simulink model "HighpassFilteredAccelerometer"  (R2019b)
settings: Solver=FixedStepAuto  StartTime=0.0  StopTime=10  FixedStep=1e-5  RelTol=1e-3
model workspace (MAT data in the model file):
  DC_Noise_Amplitude = 0.45
libraries: dsparch4 x12, simulink x9, powerlib x2
settings Model: EnablePacing=on  Creator=HUAWEI  LastModifiedBy=19398
settings DataIOCC: ReturnWorkspaceOutputs=off
settings OptimizationCC: DefaultParameterBehavior=Inlined  EnhancedBackFolding=on  PassReuseOutputArgsAs=Individual arguments  ZeroExternalMemoryAtStartup=off  ZeroInternalMemoryAtStartup=off  OptimizeBlockOrder=speed  DifferentSizesBufferReuse=on  OptimizationCustomize=off  EfficientTunableParamExpr=on
settings DebuggingCC: ParameterTunabilityLossMsg=error
settings SFSimCC: MATLABDynamicMemAlloc=off
settings RTWCC: SystemTargetFile=ert.tlc  TemplateMakefile=ert_default_tmf  GenerateReport=on  IncludeHyperlinkInReport=on  LaunchReport=on  GenerateTraceInfo=on  GenerateTraceReport=on  GenerateTraceReportSl=on  GenerateTraceReportSf=on  GenerateTraceReportEml=on
settings CodeAppCC: ForceParamTrailComments=on  IgnoreCustomStorageClasses=off  OperatorAnnotations=on  SimulinkDataObjDesc=on  SFDataObjDesc=on  InsertBlockDesc=on
settings ERTTargetCC: TargetLangStandard=C99 (ISO)  GenerateSampleERTMain=on  InlinedParameterPlacement=NonHierarchical  ERTCustomFileTemplate=example_file_process.tlc

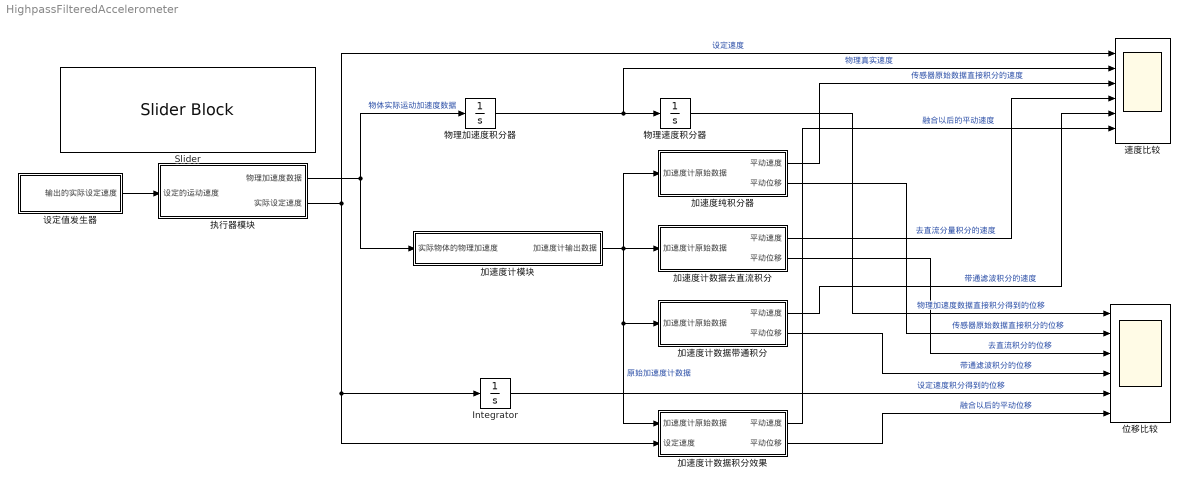
== system HighpassFilteredAccelerometer ==
  Integrator : Integrator
  Slider : SliderBlock  ScaleMin=-5  ScaleMax=5
  位移比较 : Scope  NumInputPorts=6
  加速度纯积分器 : Subsystem
  加速度计数据去直流积分 : Subsystem
  加速度计数据带通积分 : Subsystem
  加速度计数据积分效果 : Subsystem
  加速度计模块 : Subsystem
  执行器模块 : Subsystem
  物理加速度积分器 : Integrator
  物理速度积分器 : Integrator
  设定值发生器 : Subsystem
  速度比较 : Scope  NumInputPorts=6
  wires:
  执行器模块/1(物理加速度数据) -> 物理加速度积分器/1, 加速度计模块/1(实际物体的物理加速度)  "物体实际运动加速度数据"
  加速度计模块/1(加速度计输出数据) -> 加速度纯积分器/1(加速度计原始数据), 加速度计数据积分效果/1(加速度计原始数据), 加速度计数据带通积分/1(加速度计原始数据), 加速度计数据去直流积分/1(加速度计原始数据)  "原始加速度计数据"
  物理加速度积分器/1 -> 速度比较/2, 物理速度积分器/1  "物理真实速度"
  物理速度积分器/1 -> 位移比较/1  "物理加速度数据直接积分得到的位移"
  加速度纯积分器/1(平动速度) -> 速度比较/3  "传感器原始数据直接积分的速度"
  加速度计数据去直流积分/1(平动速度) -> 速度比较/4  "去直流分量积分的速度"
  加速度计数据带通积分/1(平动速度) -> 速度比较/5  "带通滤波积分的速度"
  加速度纯积分器/2(平动位移) -> 位移比较/2  "传感器原始数据直接积分的位移"
  加速度计数据去直流积分/2(平动位移) -> 位移比较/3  "去直流积分的位移"
  加速度计数据带通积分/2(平动位移) -> 位移比较/4  "带通滤波积分的位移"
  Integrator/1 -> 位移比较/5  "设定速度积分得到的位移"
  执行器模块/2(实际设定速度) -> 速度比较/1, 加速度计数据积分效果/2(设定速度), Integrator/1  "设定速度"
  加速度计数据积分效果/1(平动速度) -> 速度比较/6  "融合以后的平动速度"
  加速度计数据积分效果/2(平动位移) -> 位移比较/6  "融合以后的平动位移"
  设定值发生器/1(输出的实际设定速度) -> 执行器模块/1(设定的运动速度)

== system HighpassFilteredAccelerometer/加速度纯积分器 ==
  加速度计原始数据 : Inport
  Integrator : Integrator
  Integrator1 : Integrator
  平动速度 : Outport
  平动位移 : Outport  Port=2
  wires:
  加速度计原始数据/1 -> Integrator/1
  Integrator/1 -> Integrator1/1, 平动速度/1
  Integrator1/1 -> 平动位移/1

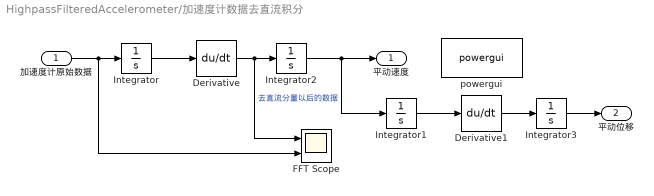
== system HighpassFilteredAccelerometer/加速度计数据去直流积分 ==
  加速度计原始数据 : Inport
  Derivative : Derivative
  Derivative1 : Derivative  CoefficientInTFapproximation=1
  "FFT Scope " : Scope  NumInputPorts=2
  Integrator{,1..3} (4 alike) : Integrator
  powergui : powerlib/powergui  Priority=1  SimulationMode=Discrete  SampleTime=1e-5  frequency=60  Iterations=50  frequencyindice=60  Pbase=100e6  ErrMax=1e-4  UnitsV=kV  UnitsW=MW  buscounter=0  FunctionMessages=off  echomessages=off  EnableUseOfTLC=off  CurrentSourceSwitches=off  DisableSnubberDevices=off  DisableRonSwitches=off  DisableVfSwitches=off  DisplayEquations=off  AutomaticDiscreteSolvers=off  SolverType=Tustin/Backward Euler (TBE)  Interpol=off  ExternalGateDelay=off  methode=off  Ts=100  x0status=blocks  SPID=on  SwTol=0  HookPort=off  NonlinearTolerance=1e-4  nMaxIteration=100  ContinueOnMaxIteration=off  RestoreLinks=warning  ResistiveCurrentMeasurement=off  Frange=[0:2:500]  Ylog=off  Xlog=on  ShowGrid=off  save=off  variable=ZData  structure=FFT_Scope1  ZoomFFT=off  StartTime=0.0  cycles=10  DisplayStyle=1  fundamental=1  FreqAxis=off  MaxFrequency=75  frequencyindicesteady=1  RmsSteady=1  display=off
      settings: SourceProductName=Simscape Electrical
  平动速度 : Outport
  平动位移 : Outport  Port=2
  wires:
  加速度计原始数据/1 -> "FFT Scope "/2, Integrator/1
  Derivative/1 -> "FFT Scope "/1, Integrator2/1  "去直流分量以后的数据"
  Derivative1/1 -> Integrator3/1
  Integrator/1 -> Derivative/1
  Integrator1/1 -> Derivative1/1
  Integrator2/1 -> Integrator1/1, 平动速度/1
  Integrator3/1 -> 平动位移/1

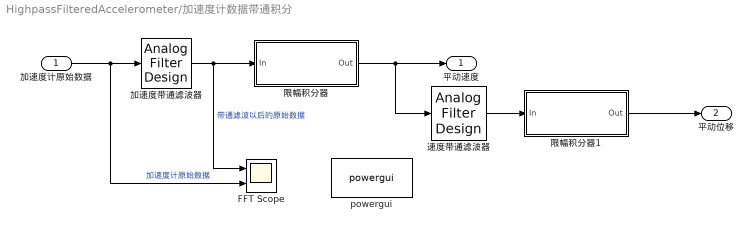
== system HighpassFilteredAccelerometer/加速度计数据带通积分 ==
  加速度计原始数据 : Inport
  FFT Scope : Scope  NumInputPorts=2
  powergui : powerlib/powergui  Priority=1  SimulationMode=Discrete  SampleTime=1e-5  frequency=60  Iterations=50  frequencyindice=60  Pbase=100e6  ErrMax=1e-4  UnitsV=kV  UnitsW=MW  buscounter=0  FunctionMessages=off  echomessages=off  EnableUseOfTLC=off  CurrentSourceSwitches=off  DisableSnubberDevices=off  DisableRonSwitches=off  DisableVfSwitches=off  DisplayEquations=off  AutomaticDiscreteSolvers=off  SolverType=Tustin/Backward Euler (TBE)  Interpol=off  ExternalGateDelay=off  methode=off  Ts=100  x0status=blocks  SPID=on  SwTol=0  HookPort=off  NonlinearTolerance=1e-4  nMaxIteration=100  ContinueOnMaxIteration=off  RestoreLinks=warning  ResistiveCurrentMeasurement=off  Frange=[0:2:500]  Ylog=off  Xlog=on  ShowGrid=off  save=off  variable=ZData  structure=FFT_Scpoe2  ZoomFFT=off  StartTime=0.0  cycles=10  DisplayStyle=1  fundamental=1  FreqAxis=off  MaxFrequency=70  frequencyindicesteady=1  RmsSteady=1  display=off
      settings: SourceProductName=Simscape Electrical
  加速度带通滤波器 : dsparch4/Analog Filter Design  method=Bessel  filttype=Bandpass  N=1  Wlo=2*pi*0.1  Whi=2*pi*300  Rp=2  Rs=40
  速度带通滤波器 : dsparch4/Analog Filter Design  method=Bessel  filttype=Bandpass  N=2  Wlo=2*pi*0.2  Whi=2*pi*300  Rp=2  Rs=40
  限幅积分器 : Subsystem
  限幅积分器1 : Subsystem
  平动速度 : Outport
  平动位移 : Outport  Port=2
  wires:
  加速度计原始数据/1 -> FFT Scope/2, 加速度带通滤波器/1  "加速度计原始数据"
  加速度带通滤波器/1 -> FFT Scope/1, 限幅积分器/1(In)  "带通滤波以后的原始数据"
  限幅积分器/1(Out) -> 平动速度/1, 速度带通滤波器/1
  速度带通滤波器/1 -> 限幅积分器1/1(In)
  限幅积分器1/1(Out) -> 平动位移/1

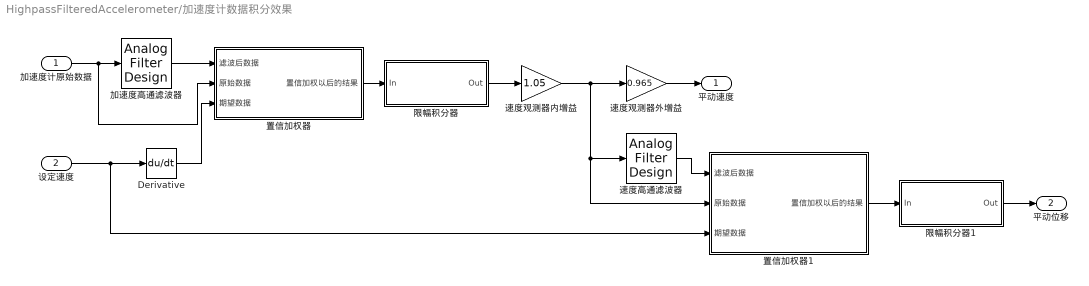
== system HighpassFilteredAccelerometer/加速度计数据积分效果 ==
  加速度计原始数据 : Inport
  设定速度 : Inport  Port=2
  Derivative : Derivative  CoefficientInTFapproximation=2
  加速度高通滤波器 : dsparch4/Analog Filter Design  method=Butterworth  filttype=Highpass  N=1  Wlo=2*pi*3  Whi=2*pi*300  Rp=2  Rs=40
  置信加权器 : Subsystem
  置信加权器1 : Subsystem
  速度观测器内增益 : Gain  Gain=1.05
  速度观测器外增益 : Gain  Gain=0.965
  速度高通滤波器 : dsparch4/Analog Filter Design  method=Butterworth  filttype=Highpass  N=1  Wlo=2*pi*5  Whi=2*pi*300  Rp=2  Rs=40
  限幅积分器 : Subsystem
  限幅积分器1 : Subsystem
  平动速度 : Outport
  平动位移 : Outport  Port=2
  wires:
  加速度计原始数据/1 -> 加速度高通滤波器/1, 置信加权器/2(原始数据)
  置信加权器/1(置信加权以后的结果) -> 限幅积分器/1(In)
  加速度高通滤波器/1 -> 置信加权器/1(滤波后数据)
  置信加权器1/1(置信加权以后的结果) -> 限幅积分器1/1(In)
  速度高通滤波器/1 -> 置信加权器1/1(滤波后数据)
  设定速度/1 -> 置信加权器1/3(期望数据), Derivative/1
  Derivative/1 -> 置信加权器/3(期望数据)
  限幅积分器/1(Out) -> 速度观测器内增益/1
  限幅积分器1/1(Out) -> 平动位移/1
  速度观测器内增益/1 -> 速度观测器外增益/1, 置信加权器1/2(原始数据), 速度高通滤波器/1
  速度观测器外增益/1 -> 平动速度/1

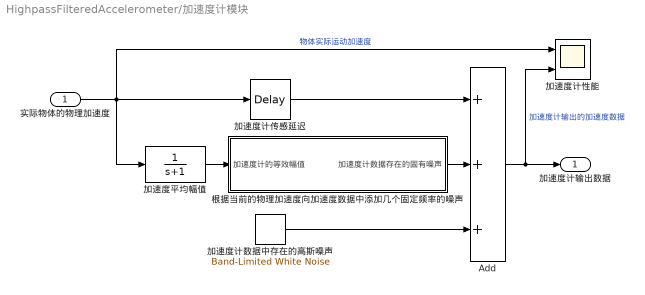
== system HighpassFilteredAccelerometer/加速度计模块 ==
  实际物体的物理加速度 : Inport
  Add : Sum  Inputs=3
  加速度平均幅值 : TransferFcn  Denominator=[1 1]
  加速度计传感延迟 : TransportDelay  DelayTime=0.0003
  加速度计性能 : Scope  NumInputPorts=2
  加速度计数据中存在的高斯噪声 : simulink/Sources/Band-Limited White Noise  Cov=[0.0000015]  Ts=0.0001  seed=[23341]
  根据当前的物理加速度向加速度数据中添加几个固定频率的噪声 : Subsystem
  加速度计输出数据 : Outport
  wires:
  根据当前的物理加速度向加速度数据中添加几个固定频率的噪声/1(加速度计数据存在的固有噪声) -> Add/2
  实际物体的物理加速度/1 -> 加速度计性能/1, 加速度计传感延迟/1, 加速度平均幅值/1  "物体实际运动加速度"
  Add/1 -> 加速度计输出数据/1, 加速度计性能/2  "加速度计输出的加速度数据"
  加速度计传感延迟/1 -> Add/1
  加速度平均幅值/1 -> 根据当前的物理加速度向加速度数据中添加几个固定频率的噪声/1(加速度计的等效幅值)
  加速度计数据中存在的高斯噪声/1 -> Add/3

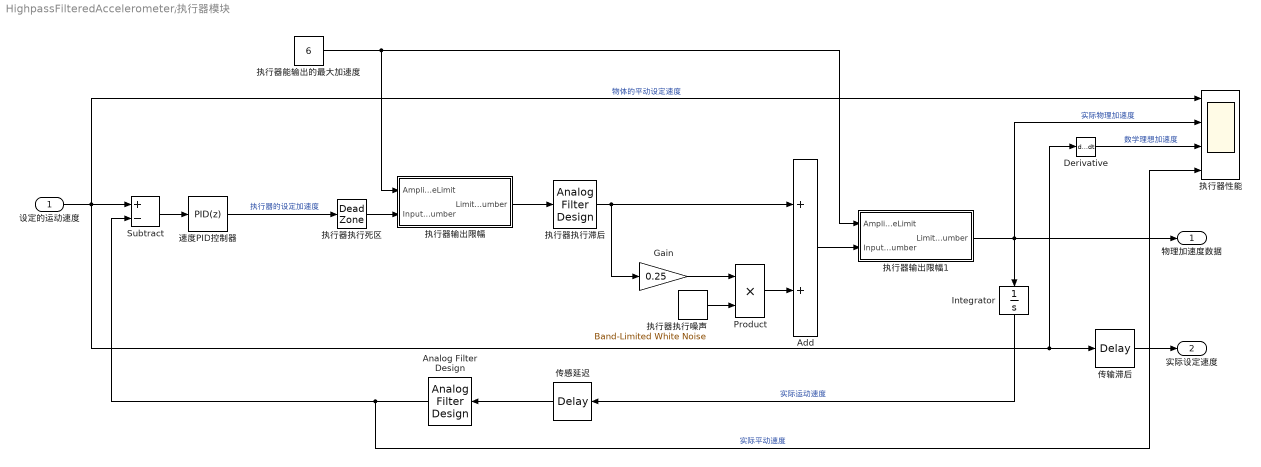
== system HighpassFilteredAccelerometer/执行器模块 ==
  设定的运动速度 : Inport
  Add : Sum
  Analog Filter Design : dsparch4/Analog Filter Design  method=Butterworth  filttype=Lowpass  N=2  Wlo=2*pi*500  Whi=80  Rp=2  Rs=40
  Derivative : Derivative
  Gain : Gain  Gain=0.25
  Integrator : Integrator
  Product : Product
  Subtract : Sum  Inputs=+-
  传感延迟 : TransportDelay  DelayTime=0.0008
  传输滞后 : TransportDelay  DelayTime=0.0003
  执行器性能 : Scope  NumInputPorts=4
  执行器执行噪声 : simulink/Sources/Band-Limited White Noise  Cov=0.0000012  Ts=0.0001  seed=[23341]
  执行器执行死区 : DeadZone  LowerValue=-0.2  UpperValue=0.2  SaturateOnIntegerOverflow=on
  执行器执行滞后 : dsparch4/Analog Filter Design  method=Butterworth  filttype=Lowpass  N=8  Wlo=2*pi*500  Whi=80  Rp=2  Rs=40
  执行器能输出的最大加速度 : Constant  Value=6
  执行器输出限幅 : Subsystem
  执行器输出限幅1 : Subsystem
  速度PID控制器 : simulink/Continuous/PID Controller  Controller=PID  Form=Parallel  TimeDomain=Discrete-time  SampleTime=0.001  IntegratorMethod=Forward Euler  FilterMethod=Forward Euler  ControllerParametersSource=internal  P=50  I=0.5  D=1  UseFilter=on  N=100  TunerSelectOption=Transfer Function Based (PID Tuner App)  InitialConditionSource=internal  InitialConditionForIntegrator=0  InitialConditionForFilter=0  DifferentiatorICPrevScaledInput=0  ExternalReset=none  TrackingMode=off  Kt=1  LimitOutput=off  UpperSaturationLimit=inf  LowerSaturationLimit=-inf  LinearizeAsGain=on  AntiWindupMode=none  Kb=1  POutMin=[]  POutMax=[]  IOutMin=[-10]  IOutMax=[10]  DOutMin=[]  DOutMax=[]  NOutMin=[]  NOutMax=[]  SumOutMin=[]  SumOutMax=[]  SaturationOutMin=[]  SaturationOutMax=[]  PParamMin=[]  PParamMax=[]  IParamMin=[]  IParamMax=[]  DParamMin=[]  DParamMax=[]  NParamMin=[]  NParamMax=[]  KbParamMin=[]  KbParamMax=[]  KtParamMin=[]  KtParamMax=[]  KbOutMin=[]  KbOutMax=[]  KtOutMin=[]  KtOutMax=[]  IntegratorOutMin=[]  IntegratorOutMax=[]  FilterOutMin=[]  FilterOutMax=[]  SumI1OutMin=[]  SumI1OutMax=[]  SumI2OutMin=[]  SumI2OutMax=[]  SumI3OutMin=[]  SumI3OutMax=[]  SumI4OutMin=[]  SumI4OutMax=[]  SumDOutMin=[]  SumDOutMax=[]  DifferentiatorOutMin=[]  DifferentiatorOutMax=[]  FilterDiffOutCoefMin=[]  FilterDiffOutCoefMax=[]  ReciprocalOutMin=[]  ReciprocalOutMax=[]  SumDenOutMin=[]  SumDenOutMax=[]  SumNumOutMin=[]  SumNumOutMax=[]  DivideOutMin=[]  DivideOutMax=[]  IntegratorContinuousStateAttributes=''  IntegratorStateMustResolveToSignalObject=off  IntegratorRTWStateStorageClass=Auto  FilterContinuousStateAttributes=''  FilterStateMustResolveToSignalObject=off  FilterRTWStateStorageClass=Auto  ParallelPVariant=InternalParameters  IdealPVariant=Disabled  IVariant=InternalParameters  DVariant=InternalParameters  IntegratorVariant=Discrete  SatVariant=Disabled  AWVariant=Passthrough  PCopyVariant=Disabled  TRVariant=Disabled  FdbkBlocksVariant=Forward  IdealPFdbkVariant=Disabled  SatFdbkVariant=Disabled  DerivativeFilterVariant=ForwardEulerFilter  NVariant=InternalParameters  NCopyVariant=Disabled  FilterICVariant=InternalICsFilter  IntegratorICVariant=InternalICs  ExternalResetVariant=Disabled  TRSumVariant=Passthrough  SumFdbkVariant=Disabled  SumVariant=Sum_PID
  物理加速度数据 : Outport
  实际设定速度 : Outport  Port=2
  wires:
  速度PID控制器/1 -> 执行器执行死区/1  "执行器的设定加速度"
  设定的运动速度/1 -> 执行器性能/1, 传输滞后/1, Derivative/1, Subtract/1  "物体的平动设定速度"
  执行器执行滞后/1 -> Gain/1, Add/1
  Derivative/1 -> 执行器性能/3  "数学理想加速度"
  传输滞后/1 -> 实际设定速度/1
  执行器输出限幅/1(LimitedNumber) -> 执行器执行滞后/1
  执行器执行死区/1 -> 执行器输出限幅/2(InputNumber)
  执行器能输出的最大加速度/1 -> 执行器输出限幅/1(AmplitudeLimit), 执行器输出限幅1/1(AmplitudeLimit)
  Product/1 -> Add/2
  执行器执行噪声/1 -> Product/2
  Gain/1 -> Product/1
  Add/1 -> 执行器输出限幅1/2(InputNumber)
  执行器输出限幅1/1(LimitedNumber) -> 执行器性能/2, 物理加速度数据/1, Integrator/1  "实际物理加速度"
  Subtract/1 -> 速度PID控制器/1
  Integrator/1 -> 传感延迟/1  "实际运动速度"
  传感延迟/1 -> Analog Filter Design/1
  Analog Filter Design/1 -> 执行器性能/4, Subtract/2  "实际平动速度"

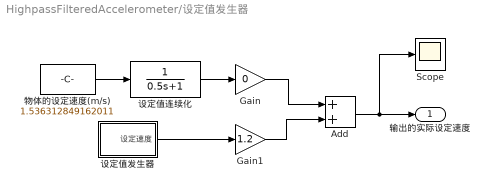
== system HighpassFilteredAccelerometer/设定值发生器 ==
  Add : Sum  Inputs=2
  Gain : Gain  Gain=0
  Gain1 : Gain  Gain=1.2
  Scope : Scope
  物体的设定速度(m/s) : Constant  Value=1.536312849162011
  设定值发生器 : Subsystem
  设定值连续化 : TransferFcn  Denominator=[0.5 1]
  输出的实际设定速度 : Outport
  wires:
  设定值发生器/1(设定速度) -> Gain1/1
  物体的设定速度(m/s)/1 -> 设定值连续化/1
  Gain1/1 -> Add/2
  设定值连续化/1 -> Gain/1
  Gain/1 -> Add/1
  Add/1 -> Scope/1, 输出的实际设定速度/1

== system HighpassFilteredAccelerometer/加速度计数据带通积分/限幅积分器 ==
  In : Inport
  Divide : Product  Inputs=**
  Integrator : Integrator
  Sign : Signum
  Square : Math  Operator=square  SignedPower=off  SaturateOnIntegerOverflow=on
  Switch : Switch  Criteria=u2 > Threshold  Threshold=0.3
  Out : Outport
  wires:
  Integrator/1 -> Out/1
  In/1 -> Switch/1, Sign/1, Square/1, Switch/2
  Switch/1 -> Integrator/1
  Square/1 -> Divide/1
  Sign/1 -> Divide/2
  Divide/1 -> Switch/3

== system HighpassFilteredAccelerometer/加速度计数据带通积分/限幅积分器1 ==
  In : Inport
  Divide : Product  Inputs=**
  Integrator : Integrator
  Sign : Signum
  Square : Math  Operator=square  SignedPower=off  SaturateOnIntegerOverflow=on
  Switch : Switch  Criteria=u2 > Threshold  Threshold=0.3
  Out : Outport
  wires:
  In/1 -> Switch/1, Sign/1, Square/1, Switch/2
  Integrator/1 -> Out/1
  Square/1 -> Divide/1
  Sign/1 -> Divide/2
  Divide/1 -> Switch/3
  Switch/1 -> Integrator/1

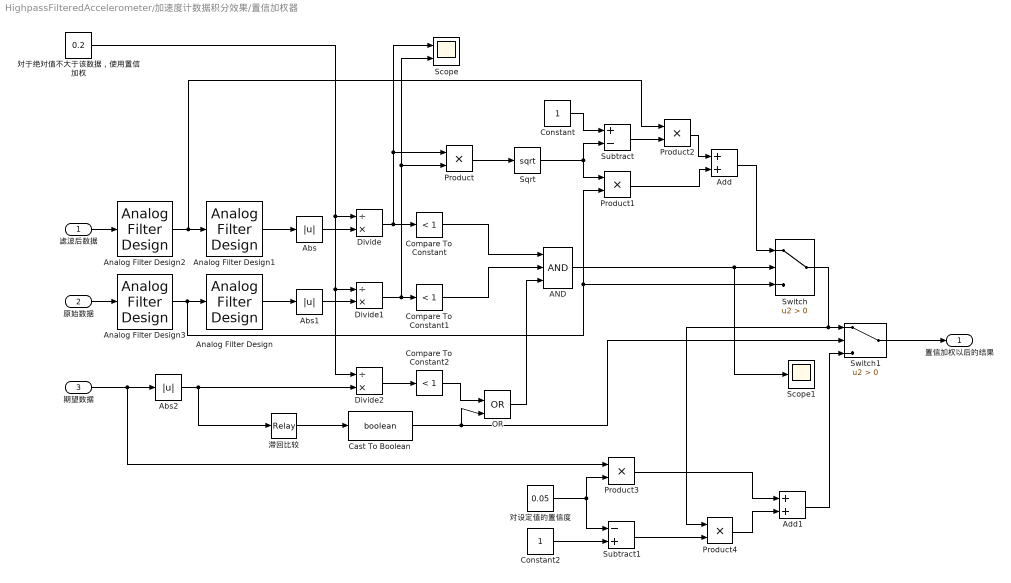
== system HighpassFilteredAccelerometer/加速度计数据积分效果/置信加权器 ==
  滤波后数据 : Inport
  原始数据 : Inport  Port=2
  期望数据 : Inport  Port=3
  AND : Logic  Inputs=3  IconShape=distinctive  AllPortsSameDT=off  OutDataTypeStr=boolean
  Abs : Abs
  Abs1 : Abs
  Abs2 : Abs
  Add : Sum
  Add1 : Sum
  Analog Filter Design : dsparch4/Analog Filter Design  method=Butterworth  filttype=Lowpass  N=2  Wlo=2*pi*10  Whi=2*pi*80  Rp=2  Rs=40
  Analog Filter Design1 : dsparch4/Analog Filter Design  method=Butterworth  filttype=Lowpass  N=2  Wlo=2*pi*10  Whi=2*pi*80  Rp=2  Rs=40
  Analog Filter Design2 : dsparch4/Analog Filter Design  method=Butterworth  filttype=Lowpass  N=1  Wlo=2*pi*150  Whi=80  Rp=2  Rs=40
  Analog Filter Design3 : dsparch4/Analog Filter Design  method=Butterworth  filttype=Lowpass  N=1  Wlo=2*pi*150  Whi=80  Rp=2  Rs=40
  Cast To Boolean : DataTypeConversion  OutDataTypeStr=boolean
  Compare To Constant : simulink/Logic and Bit Operations/Compare To Constant  relop=<  const=1  OutDataTypeStr=boolean
  Compare To Constant1 : simulink/Logic and Bit Operations/Compare To Constant  relop=<  const=1  OutDataTypeStr=boolean
  Compare To Constant2 : simulink/Logic and Bit Operations/Compare To Constant  relop=<  const=1  OutDataTypeStr=boolean
  Constant : Constant
  Constant2 : Constant
  Divide : Product  Inputs=/*
  Divide1 : Product  Inputs=/*
  Divide2 : Product  Inputs=/*
  OR : Logic  Operator=OR  IconShape=distinctive  AllPortsSameDT=off  OutDataTypeStr=boolean
  Product{,1..4} (5 alike) : Product
  Scope : Scope  NumInputPorts=2
  Scope1 : Scope
  Sqrt : Sqrt  SaturateOnIntegerOverflow=on
  Subtract : Sum  Inputs=+-
  Subtract1 : Sum  Inputs=-+
  Switch : Switch  Criteria=u2 > Threshold
  Switch1 : Switch  Criteria=u2 > Threshold
  对于绝对值不大于该数据，使用置信加权 : Constant  Value=0.2
  对设定值的置信度 : Constant  Value=0.05
  滞回比较 : Relay  OnSwitchValue=3  OffSwitchValue=1
  置信加权以后的结果 : Outport
  wires:
  滤波后数据/1 -> Analog Filter Design2/1
  原始数据/1 -> Analog Filter Design3/1
  Abs/1 -> Divide/2
  对于绝对值不大于该数据，使用置信加权/1 -> Divide2/1, Divide1/1, Divide/1
  Abs1/1 -> Divide1/2
  Divide/1 -> Scope/1, Product/1, Compare To Constant/1
  Divide1/1 -> Scope/2, Product/2, Compare To Constant1/1
  Compare To Constant/1 -> AND/1
  Compare To Constant1/1 -> AND/2
  AND/1 -> Scope1/1, Switch/2
  Constant/1 -> Subtract/1
  Product/1 -> Sqrt/1
  Subtract/1 -> Product2/2
  Product2/1 -> Add/1
  Product1/1 -> Add/2
  Add/1 -> Switch/1
  Sqrt/1 -> Product1/1, Subtract/2
  Analog Filter Design/1 -> Abs1/1
  期望数据/1 -> Product3/1, Abs2/1
  Abs2/1 -> 滞回比较/1, Divide2/2
  Divide2/1 -> Compare To Constant2/1
  Analog Filter Design1/1 -> Abs/1
  Compare To Constant2/1 -> OR/1
  OR/1 -> AND/3
  滞回比较/1 -> Cast To Boolean/1
  Cast To Boolean/1 -> Switch1/2, OR/2
  Switch/1 -> Product4/1, Switch1/1
  Switch1/1 -> 置信加权以后的结果/1
  对设定值的置信度/1 -> Product3/2, Subtract1/1
  Constant2/1 -> Subtract1/2
  Subtract1/1 -> Product4/2
  Product3/1 -> Add1/1
  Product4/1 -> Add1/2
  Analog Filter Design2/1 -> Analog Filter Design1/1, Product2/1
  Analog Filter Design3/1 -> Analog Filter Design/1, Product1/2, Switch/3
  Add1/1 -> Switch1/3

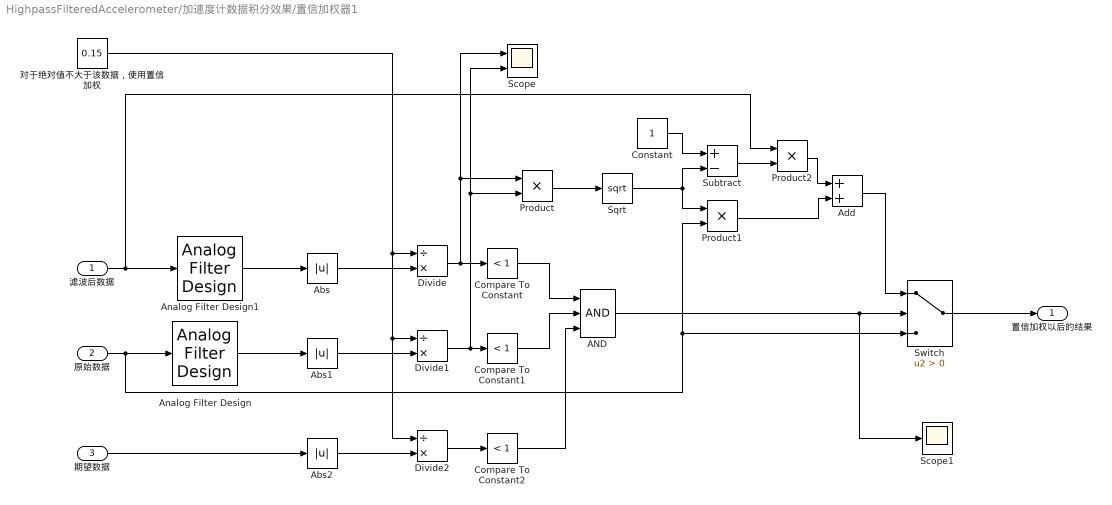
== system HighpassFilteredAccelerometer/加速度计数据积分效果/置信加权器1 ==
  滤波后数据 : Inport
  原始数据 : Inport  Port=2
  期望数据 : Inport  Port=3
  AND : Logic  Inputs=3  IconShape=distinctive  AllPortsSameDT=off  OutDataTypeStr=boolean
  Abs : Abs
  Abs1 : Abs
  Abs2 : Abs
  Add : Sum
  Analog Filter Design : dsparch4/Analog Filter Design  method=Butterworth  filttype=Lowpass  N=8  Wlo=2*pi*20  Whi=80  Rp=2  Rs=40
  Analog Filter Design1 : dsparch4/Analog Filter Design  method=Butterworth  filttype=Lowpass  N=8  Wlo=2*pi*20  Whi=80  Rp=2  Rs=40
  Compare To Constant : simulink/Logic and Bit Operations/Compare To Constant  relop=<  const=1  OutDataTypeStr=boolean
  Compare To Constant1 : simulink/Logic and Bit Operations/Compare To Constant  relop=<  const=1  OutDataTypeStr=boolean
  Compare To Constant2 : simulink/Logic and Bit Operations/Compare To Constant  relop=<  const=1  OutDataTypeStr=boolean
  Constant : Constant
  Divide : Product  Inputs=/*
  Divide1 : Product  Inputs=/*
  Divide2 : Product  Inputs=/*
  Product : Product
  Product1 : Product
  Product2 : Product
  Scope : Scope  NumInputPorts=2
  Scope1 : Scope
  Sqrt : Sqrt  SaturateOnIntegerOverflow=on
  Subtract : Sum  Inputs=+-
  Switch : Switch  Criteria=u2 > Threshold
  对于绝对值不大于该数据，使用置信加权 : Constant  Value=0.15
  置信加权以后的结果 : Outport
  wires:
  滤波后数据/1 -> Analog Filter Design1/1, Product2/1
  原始数据/1 -> Analog Filter Design/1, Product1/2, Switch/3
  Abs/1 -> Divide/2
  对于绝对值不大于该数据，使用置信加权/1 -> Divide2/1, Divide1/1, Divide/1
  Abs1/1 -> Divide1/2
  Divide/1 -> Scope/1, Product/1, Compare To Constant/1
  Divide1/1 -> Scope/2, Product/2, Compare To Constant1/1
  Compare To Constant/1 -> AND/1
  Compare To Constant1/1 -> AND/2
  AND/1 -> Scope1/1, Switch/2
  Switch/1 -> 置信加权以后的结果/1
  Constant/1 -> Subtract/1
  Product/1 -> Sqrt/1
  Subtract/1 -> Product2/2
  Product2/1 -> Add/1
  Product1/1 -> Add/2
  Add/1 -> Switch/1
  Sqrt/1 -> Product1/1, Subtract/2
  Analog Filter Design/1 -> Abs1/1
  期望数据/1 -> Abs2/1
  Abs2/1 -> Divide2/2
  Divide2/1 -> Compare To Constant2/1
  Compare To Constant2/1 -> AND/3
  Analog Filter Design1/1 -> Abs/1

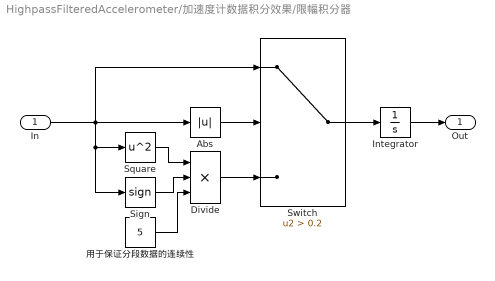
== system HighpassFilteredAccelerometer/加速度计数据积分效果/限幅积分器 ==
  In : Inport
  Abs : Abs
  Divide : Product  Inputs=***
  Integrator : Integrator
  Sign : Signum
  Square : Math  Operator=square  SignedPower=off  SaturateOnIntegerOverflow=on
  Switch : Switch  Criteria=u2 > Threshold  Threshold=0.2
  用于保证分段数据的连续性 : Constant  Value=5
  Out : Outport
  wires:
  Integrator/1 -> Out/1
  In/1 -> Switch/1, Sign/1, Square/1, Abs/1
  Switch/1 -> Integrator/1
  Square/1 -> Divide/1
  Sign/1 -> Divide/2
  Divide/1 -> Switch/3
  Abs/1 -> Switch/2
  用于保证分段数据的连续性/1 -> Divide/3

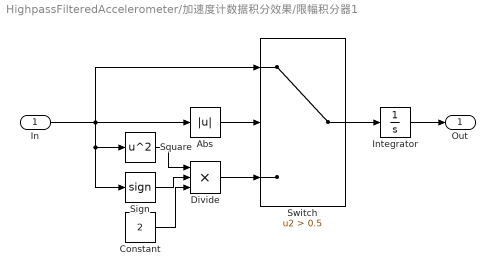
== system HighpassFilteredAccelerometer/加速度计数据积分效果/限幅积分器1 ==
  In : Inport
  Abs : Abs
  Constant : Constant  Value=2
  Divide : Product  Inputs=***
  Integrator : Integrator
  Sign : Signum
  Square : Math  Operator=square  SignedPower=off  SaturateOnIntegerOverflow=on
  Switch : Switch  Criteria=u2 > Threshold  Threshold=0.5
  Out : Outport
  wires:
  Integrator/1 -> Out/1
  In/1 -> Switch/1, Sign/1, Square/1, Abs/1
  Switch/1 -> Integrator/1
  Square/1 -> Divide/1
  Sign/1 -> Divide/2
  Divide/1 -> Switch/3
  Abs/1 -> Switch/2
  Constant/1 -> Divide/3

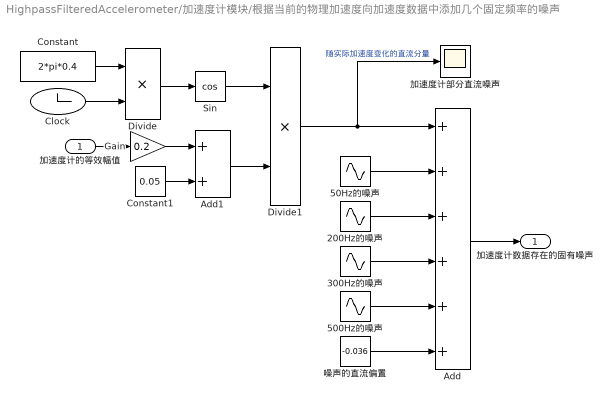
== system HighpassFilteredAccelerometer/加速度计模块/根据当前的物理加速度向加速度数据中添加几个固定频率的噪声 ==
  加速度计的等效幅值 : Inport
  200Hz的噪声 : Sin  Amplitude=0.1  Frequency=2*pi*200  SampleTime=0
  300Hz的噪声 : Sin  Amplitude=0.06  Frequency=2*pi*300  Phase=0.1*pi  SampleTime=0
  500Hz的噪声 : Sin  Amplitude=0.05  Frequency=2*pi*500  Phase=0.3*pi  SampleTime=0
  50Hz的噪声 : Sin  Amplitude=0.18  Frequency=2*pi*50  Phase=-0.3*pi  SampleTime=0
  Add : Sum  Inputs=++++++
  Add1 : Sum
  Clock : Clock
      settings: Decimation=100000
  Constant : Constant  Value=2*pi*0.4
  Constant1 : Constant  Value=0.05
  Divide : Product  Inputs=**
  Divide1 : Product  Inputs=**
  Gain : Gain  Gain=0.2
  Sin : Trigonometry  Operator=cos
  加速度计部分直流噪声 : Scope
  噪声的直流偏置 : Constant  Value=-0.036
  加速度计数据存在的固有噪声 : Outport
  wires:
  300Hz的噪声/1 -> Add/4
  200Hz的噪声/1 -> Add/3
  50Hz的噪声/1 -> Add/2
  500Hz的噪声/1 -> Add/5
  Add/1 -> 加速度计数据存在的固有噪声/1
  Clock/1 -> Divide/2
  Divide/1 -> Sin/1
  Constant/1 -> Divide/1
  Sin/1 -> Divide1/1
  加速度计的等效幅值/1 -> Gain/1
  Divide1/1 -> 加速度计部分直流噪声/1, Add/1  "随实际加速度变化的直流分量"
  Gain/1 -> Add1/1
  Add1/1 -> Divide1/2
  Constant1/1 -> Add1/2
  噪声的直流偏置/1 -> Add/6

== system HighpassFilteredAccelerometer/执行器模块/执行器输出限幅 ==
  AmplitudeLimit : Inport
  InputNumber : Inport  Port=2
  Abs : Abs
  Max : MinMax  Inputs=2
  Max1 : MinMax  Function=max  Inputs=2
  Minus : Sum  Inputs=-
  LimitedNumber : Outport
  wires:
  AmplitudeLimit/1 -> Abs/1
  Max1/1 -> LimitedNumber/1
  InputNumber/1 -> Max/1
  Abs/1 -> Minus/1, Max/2
  Minus/1 -> Max1/1
  Max/1 -> Max1/2

== system HighpassFilteredAccelerometer/执行器模块/执行器输出限幅1 ==
  AmplitudeLimit : Inport
  InputNumber : Inport  Port=2
  Abs : Abs
  Max : MinMax  Inputs=2
  Max1 : MinMax  Function=max  Inputs=2
  Minus : Sum  Inputs=-
  LimitedNumber : Outport
  wires:
  AmplitudeLimit/1 -> Abs/1
  Max1/1 -> LimitedNumber/1
  InputNumber/1 -> Max/1
  Abs/1 -> Minus/1, Max/2
  Max/1 -> Max1/2
  Minus/1 -> Max1/1

== system HighpassFilteredAccelerometer/设定值发生器/设定值发生器 ==
  Scope : Scope
  Sine Wave : Sin  Amplitude=3  Frequency=2*pi*0.2  SampleTime=0
  设定速度 : Outport
  wires:
  Sine Wave/1 -> 设定速度/1, Scope/1
